simulink library "AEMACE10_OUT"  (R2021b)
settings: Solver=VariableStepAuto  StartTime=0.0  StopTime=10.0  RelTol=1e-3
settings Model: Creator=ACH  LastModifiedBy=ACH

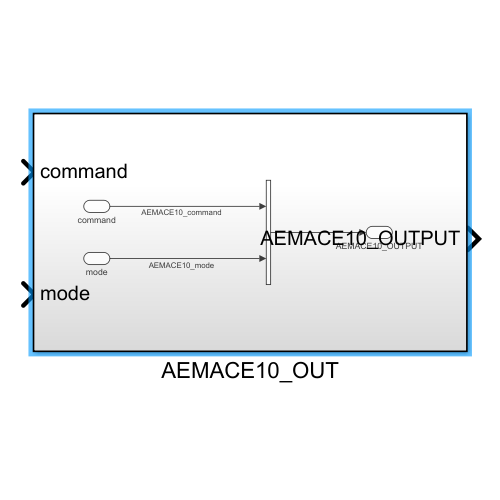
[thumbnail: Simulink's stored preview of the top-level diagram]
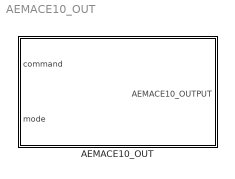
== system AEMACE10_OUT ==
  AEMACE10_OUT : Subsystem

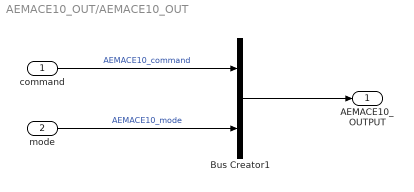
== system AEMACE10_OUT/AEMACE10_OUT ==
  command : Inport
  mode : Inport  Port=2
  Bus Creator1 : BusCreator  Inputs=2  OutDataTypeStr=Bus: AEMACE10_OUTPUT
  AEMACE10_OUTPUT : Outport  OutDataTypeStr=Bus: AEMACE10_OUTPUT
  wires:
  command/1 -> Bus Creator1/1  "AEMACE10_command"
  mode/1 -> Bus Creator1/2  "AEMACE10_mode"
  Bus Creator1/1 -> AEMACE10_OUTPUT/1
